simulink subsystem "window_control"  (R2021b)
settings: Solver=VariableStepAuto  StartTime=0.0  StopTime=10.0  RelTol=1e-3
values from neighbouring files (symbols this model uses):
  armature_position = Simulink.Parameter    [Parameters.m]
  energy_save_speed = Simulink.Parameter    [Parameters.m]
  window_speed = Simulink.Parameter    [Parameters.m]
libraries: simulink x1
settings Model: Creator=Mindmotiv  LastModifiedBy=wiechowski
settings SolverCC: AlgebraicLoopSolver=TrustRegion
settings DebuggingCC: SFMachineParentedDataDiag=warning

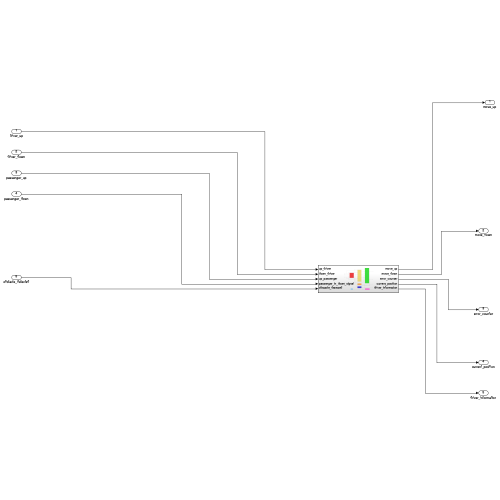
[thumbnail: Simulink's stored preview of the top-level diagram]
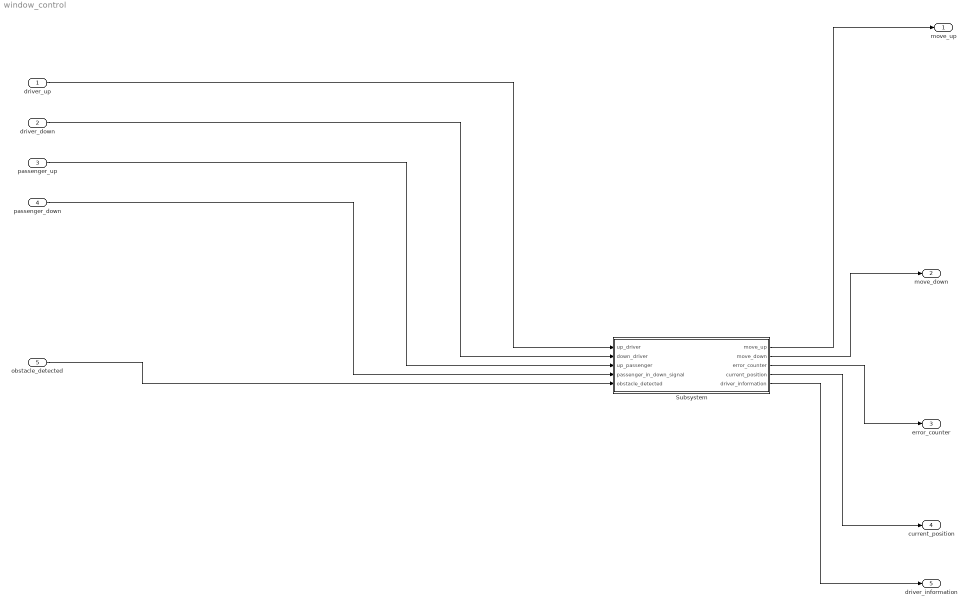
== system window_control ==
  driver_up : Inport
  driver_down : Inport  Port=2
  passenger_up : Inport  Port=3
  passenger_down : Inport  Port=4
  obstacle_detected : Inport  Port=5
  Subsystem : Subsystem
  move_up : Outport
  move_down : Outport  Port=2
  error_counter : Outport  Port=3
  current_position : Outport  Port=4
  driver_information : Outport  Port=5
  wires:
  driver_up/1 -> Subsystem/1(up_driver)
  driver_down/1 -> Subsystem/2(down_driver)
  passenger_up/1 -> Subsystem/3(up_passenger)
  passenger_down/1 -> Subsystem/4(passenger_in_down_signal)
  obstacle_detected/1 -> Subsystem/5(obstacle_detected)
  Subsystem/1(move_up) -> move_up/1
  Subsystem/2(move_down) -> move_down/1
  Subsystem/3(error_counter) -> error_counter/1
  Subsystem/4(current_position) -> current_position/1
  Subsystem/5(driver_information) -> driver_information/1

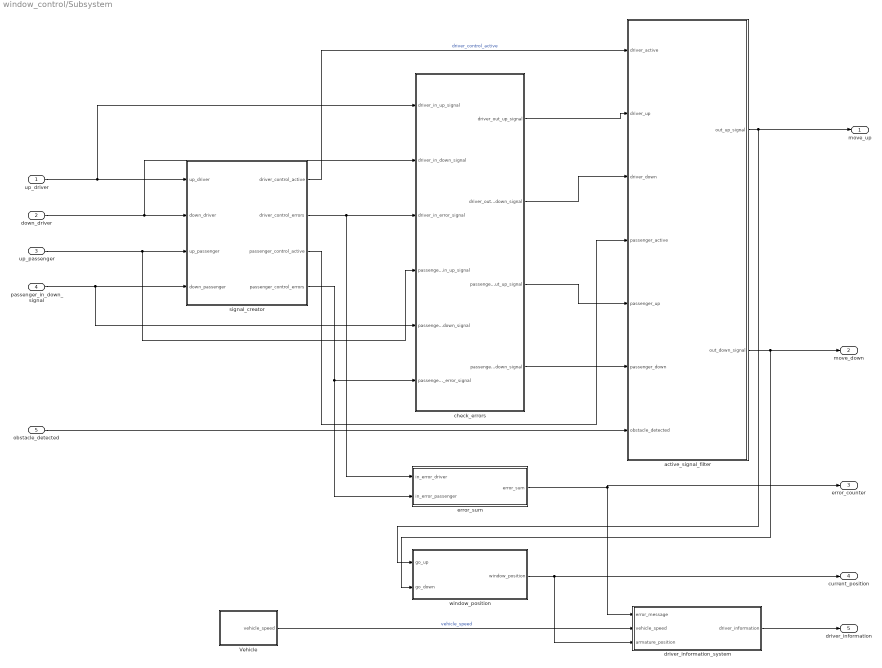
== system window_control/Subsystem ==
  up_driver : Inport
  down_driver : Inport  Port=2
  up_passenger : Inport  Port=3
  passenger_in_down_signal : Inport  Port=4
  obstacle_detected : Inport  Port=5
  Vehicle : Subsystem
  active_signal_filter : Subsystem
  check_errors : Subsystem
  driver_information_system : Subsystem
  error_sum : Subsystem
  signal_creator : Subsystem
  window_position : Subsystem
  move_up : Outport
  move_down : Outport  Port=2
  error_counter : Outport  Port=3
  current_position : Outport  Port=4
  driver_information : Outport  Port=5
  wires:
  obstacle_detected/1 -> active_signal_filter/7(obstacle_detected)
  check_errors/2(driver_out_down_signal) -> active_signal_filter/3(driver_down)
  driver_information_system/1(driver_information) -> driver_information/1
  Vehicle/1(vehicle_speed) -> driver_information_system/2(vehicle_speed)  "vehicle_speed"
  signal_creator/3(passenger_control_active) -> active_signal_filter/4(passenger_active)
  signal_creator/1(driver_control_active) -> active_signal_filter/1(driver_active)  "driver_control_active"
  check_errors/3(passenger_out_up_signal) -> active_signal_filter/5(passenger_up)
  check_errors/4(passenger_out_down_signal) -> active_signal_filter/6(passenger_down)
  up_passenger/1 -> signal_creator/3(up_passenger), check_errors/4(passenger_in_up_signal)
  window_position/1(window_position) -> current_position/1, driver_information_system/3(armature_position)
  up_driver/1 -> signal_creator/1(up_driver), check_errors/1(driver_in_up_signal)
  down_driver/1 -> signal_creator/2(down_driver), check_errors/2(driver_in_down_signal)
  signal_creator/4(passenger_control_errors) -> check_errors/6(passenger_in_error_signal), error_sum/2(in_error_passenger)
  passenger_in_down_signal/1 -> check_errors/5(passenger_in_down_signal), signal_creator/4(down_passenger)
  signal_creator/2(driver_control_errors) -> check_errors/3(driver_in_error_signal), error_sum/1(in_error_driver)
  active_signal_filter/1(out_up_signal) -> move_up/1, window_position/1(go_up)
  check_errors/1(driver_out_up_signal) -> active_signal_filter/2(driver_up)
  active_signal_filter/2(out_down_signal) -> move_down/1, window_position/2(go_down)
  error_sum/1(error_sum) -> error_counter/1, driver_information_system/1(error_message)

== system window_control/Subsystem/Vehicle ==
  Constant : Constant  Value=0
  vehicle_speed : Outport
  wires:
  Constant/1 -> vehicle_speed/1

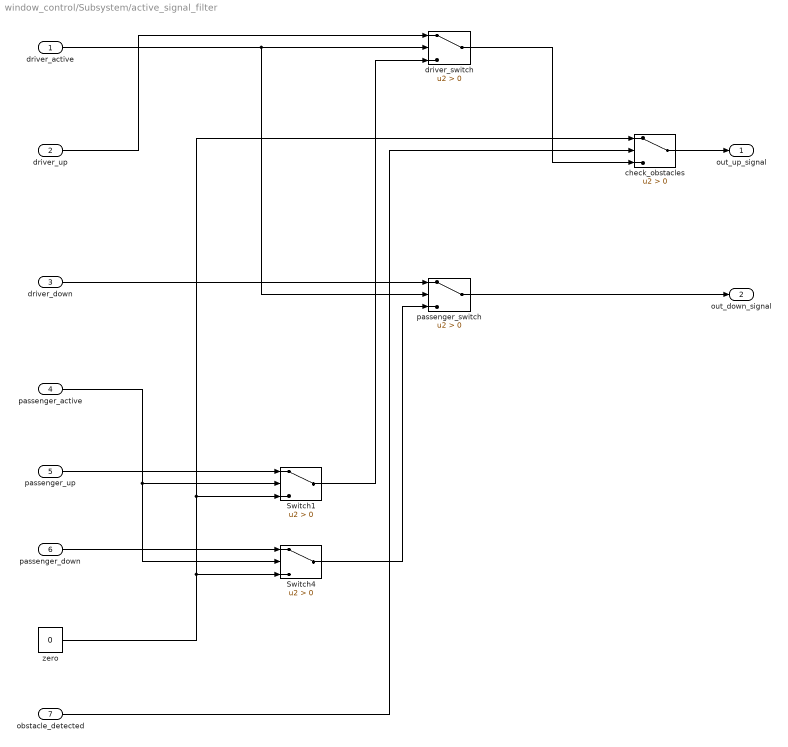
== system window_control/Subsystem/active_signal_filter ==
  driver_active : Inport
  driver_up : Inport  Port=2
  driver_down : Inport  Port=3
  passenger_active : Inport  Port=4
  passenger_up : Inport  Port=5
  passenger_down : Inport  Port=6
  obstacle_detected : Inport  Port=7
  Switch1 : Switch  Criteria=u2 > Threshold
  Switch4 : Switch  Criteria=u2 > Threshold
  check_obstacles : Switch  Criteria=u2 > Threshold
  driver_switch : Switch  Criteria=u2 > Threshold
  passenger_switch : Switch  Criteria=u2 > Threshold
  zero : Constant  Value=0
  out_up_signal : Outport
  out_down_signal : Outport  Port=2
  wires:
  check_obstacles/1 -> out_up_signal/1
  driver_switch/1 -> check_obstacles/3
  obstacle_detected/1 -> check_obstacles/2
  passenger_switch/1 -> out_down_signal/1
  Switch4/1 -> passenger_switch/3
  passenger_down/1 -> Switch4/1
  driver_down/1 -> passenger_switch/1
  passenger_up/1 -> Switch1/1
  Switch1/1 -> driver_switch/3
  passenger_active/1 -> Switch1/2, Switch4/2
  driver_up/1 -> driver_switch/1
  zero/1 -> Switch1/3, check_obstacles/1, Switch4/3
  driver_active/1 -> driver_switch/2, passenger_switch/2

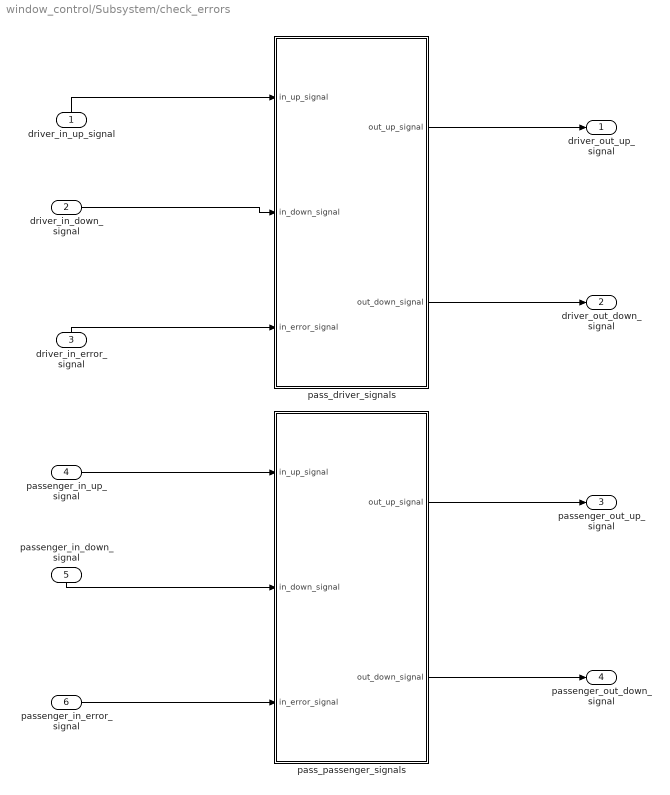
== system window_control/Subsystem/check_errors ==
  driver_in_up_signal : Inport
  driver_in_down_signal : Inport  Port=2
  driver_in_error_signal : Inport  Port=3
  passenger_in_up_signal : Inport  Port=4
  passenger_in_down_signal : Inport  Port=5
  passenger_in_error_signal : Inport  Port=6
  pass_driver_signals : Subsystem
  pass_passenger_signals : Subsystem
  driver_out_up_signal : Outport
  driver_out_down_signal : Outport  Port=2
  passenger_out_up_signal : Outport  Port=3
  passenger_out_down_signal : Outport  Port=4
  wires:
  driver_in_error_signal/1 -> pass_driver_signals/3(in_error_signal)
  pass_driver_signals/2(out_down_signal) -> driver_out_down_signal/1
  pass_driver_signals/1(out_up_signal) -> driver_out_up_signal/1
  passenger_in_error_signal/1 -> pass_passenger_signals/3(in_error_signal)
  passenger_in_down_signal/1 -> pass_passenger_signals/2(in_down_signal)
  driver_in_down_signal/1 -> pass_driver_signals/2(in_down_signal)
  passenger_in_up_signal/1 -> pass_passenger_signals/1(in_up_signal)
  pass_passenger_signals/1(out_up_signal) -> passenger_out_up_signal/1
  driver_in_up_signal/1 -> pass_driver_signals/1(in_up_signal)
  pass_passenger_signals/2(out_down_signal) -> passenger_out_down_signal/1

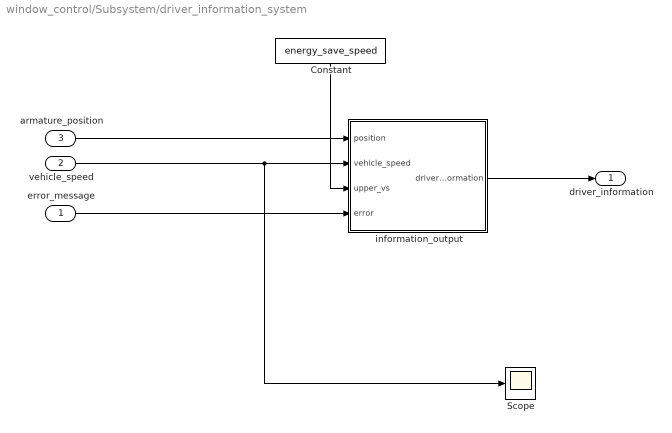
== system window_control/Subsystem/driver_information_system ==
  error_message : Inport
  vehicle_speed : Inport  Port=2
  armature_position : Inport  Port=3
  Constant : Constant  Value=energy_save_speed
  Scope : Scope
  information_output : MATLAB Function  TreatAsAtomicUnit=on
  driver_information : Outport
  wires:
  armature_position/1 -> information_output/1(position)
  information_output/1(driver_information) -> driver_information/1
  vehicle_speed/1 -> information_output/2(vehicle_speed), Scope/1
  error_message/1 -> information_output/4(error)
  Constant/1 -> information_output/3(upper_vs)

== system window_control/Subsystem/error_sum ==
  in_error_driver : Inport
  in_error_passenger : Inport  Port=2
  Add : Sum
  error_sum : Outport
  wires:
  in_error_driver/1 -> Add/1
  in_error_passenger/1 -> Add/2
  Add/1 -> error_sum/1

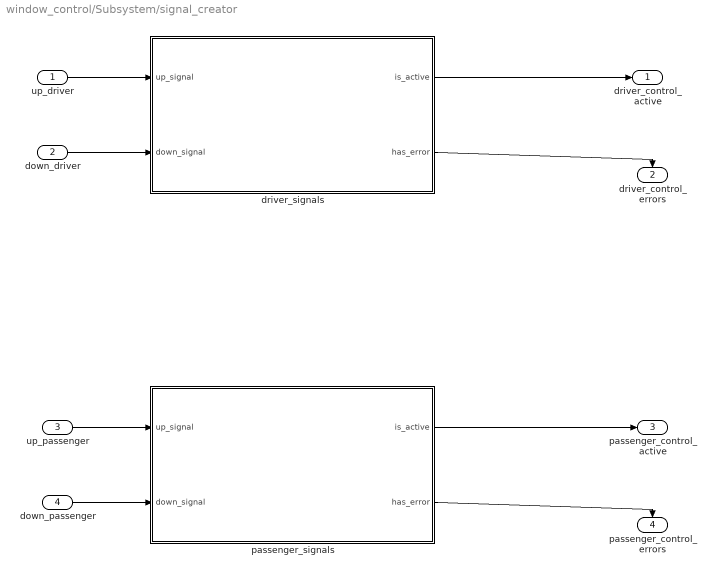
== system window_control/Subsystem/signal_creator ==
  up_driver : Inport
  down_driver : Inport  Port=2
  up_passenger : Inport  Port=3
  down_passenger : Inport  Port=4
  driver_signals : Subsystem
  passenger_signals : Subsystem
  driver_control_active : Outport
  driver_control_errors : Outport  Port=2
  passenger_control_active : Outport  Port=3
  passenger_control_errors : Outport  Port=4
  wires:
  up_passenger/1 -> passenger_signals/1(up_signal)
  up_driver/1 -> driver_signals/1(up_signal)
  down_passenger/1 -> passenger_signals/2(down_signal)
  passenger_signals/2(has_error) -> passenger_control_errors/1
  down_driver/1 -> driver_signals/2(down_signal)
  passenger_signals/1(is_active) -> passenger_control_active/1
  driver_signals/2(has_error) -> driver_control_errors/1
  driver_signals/1(is_active) -> driver_control_active/1

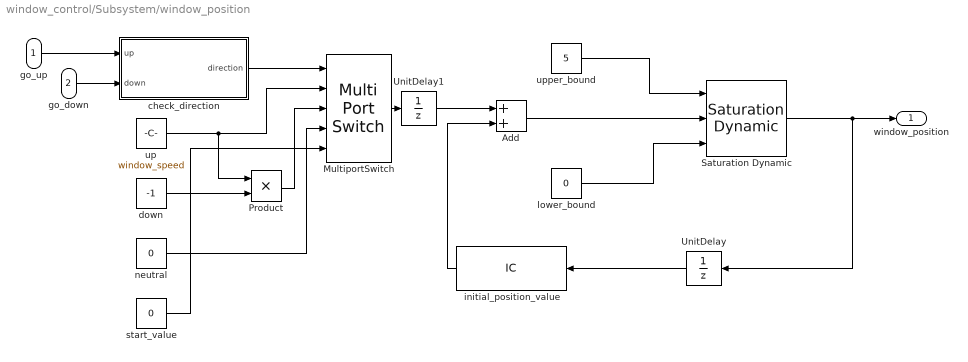
== system window_control/Subsystem/window_position ==
  go_up : Inport
  go_down : Inport  Port=2
  Add : Sum
  MultiportSwitch : MultiPortSwitch  DataPortOrder=Zero-based contiguous  Inputs=4  zeroidx=on
  Product : Product  RndMeth=Zero
  Saturation Dynamic : simulink/Discontinuities/Saturation Dynamic  OutMin=0  OutMax=100  OutDataTypeStr=Inherit: Same as second input  OutDataType=fixdt(1, 16)  OutScaling=2^-10  DoSatur=off
  UnitDelay : UnitDelay  SampleTime=-1  HasFrameUpgradeWarning=on
  UnitDelay1 : UnitDelay  SampleTime=-1  HasFrameUpgradeWarning=on
  check_direction : MATLAB Function  TreatAsAtomicUnit=on
  down : Constant  Value=-1
  initial_position_value : InitialCondition  Value=armature_position
  lower_bound : Constant  Value=0
  neutral : Constant  Value=0
  start_value : Constant  Value=0
  up : Constant  Value=window_speed
  upper_bound : Constant  Value=5
  window_position : Outport
  wires:
  UnitDelay1/1 -> Add/1
  Product/1 -> MultiportSwitch/3
  Add/1 -> Saturation Dynamic/2
  up/1 -> MultiportSwitch/2, Product/1
  start_value/1 -> MultiportSwitch/5
  Saturation Dynamic/1 -> window_position/1, UnitDelay/1
  check_direction/1(direction) -> MultiportSwitch/1
  down/1 -> Product/2
  neutral/1 -> MultiportSwitch/4
  MultiportSwitch/1 -> UnitDelay1/1
  go_up/1 -> check_direction/1(up)
  UnitDelay/1 -> initial_position_value/1
  lower_bound/1 -> Saturation Dynamic/3
  go_down/1 -> check_direction/2(down)
  initial_position_value/1 -> Add/2
  upper_bound/1 -> Saturation Dynamic/1

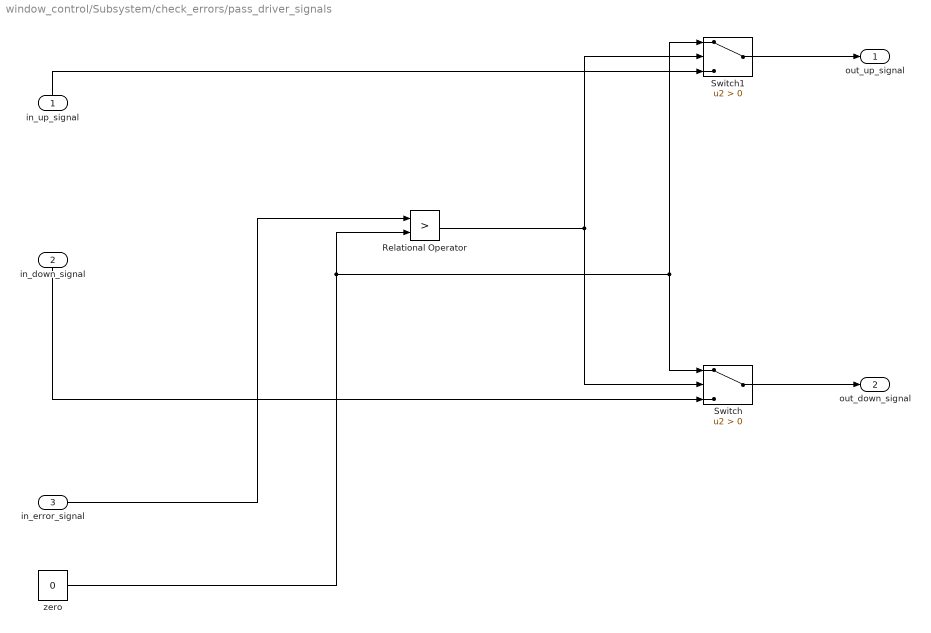
== system window_control/Subsystem/check_errors/pass_driver_signals ==
  in_up_signal : Inport
  in_down_signal : Inport  Port=2
  in_error_signal : Inport  Port=3
  Relational Operator : RelationalOperator  Operator=>  OutDataTypeStr=boolean  RndMeth=Nearest
  Switch : Switch  Criteria=u2 > Threshold
  Switch1 : Switch  Criteria=u2 > Threshold
  zero : Constant  Value=0
  out_up_signal : Outport
  out_down_signal : Outport  Port=2
  wires:
  Relational Operator/1 -> Switch/2, Switch1/2
  Switch/1 -> out_down_signal/1
  zero/1 -> Relational Operator/2, Switch/1, Switch1/1
  in_error_signal/1 -> Relational Operator/1
  in_down_signal/1 -> Switch/3
  in_up_signal/1 -> Switch1/3
  Switch1/1 -> out_up_signal/1

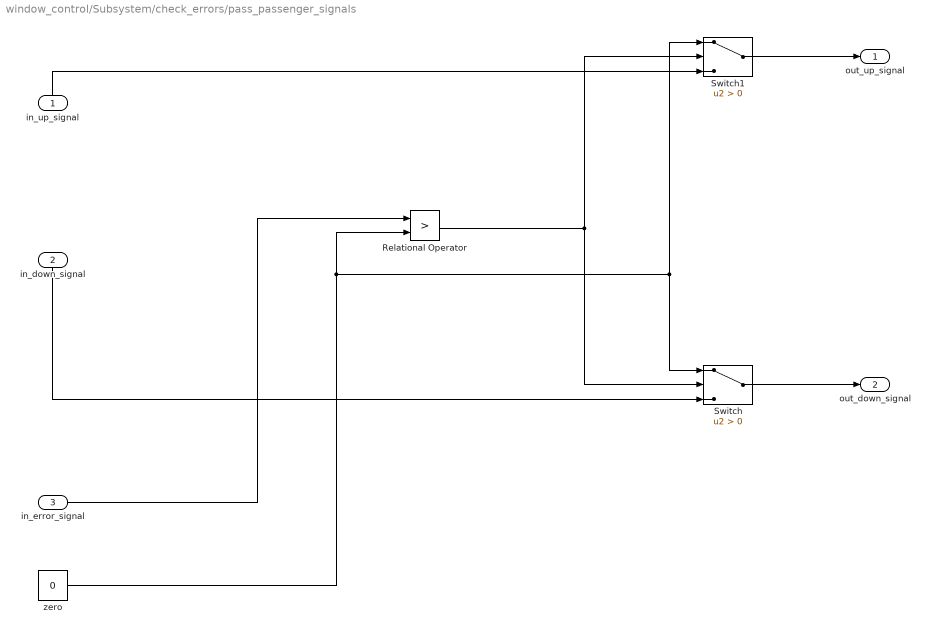
== system window_control/Subsystem/check_errors/pass_passenger_signals ==
  in_up_signal : Inport
  in_down_signal : Inport  Port=2
  in_error_signal : Inport  Port=3
  Relational Operator : RelationalOperator  Operator=>  OutDataTypeStr=boolean  RndMeth=Nearest
  Switch : Switch  Criteria=u2 > Threshold
  Switch1 : Switch  Criteria=u2 > Threshold
  zero : Constant  Value=0
  out_up_signal : Outport
  out_down_signal : Outport  Port=2
  wires:
  Relational Operator/1 -> Switch/2, Switch1/2
  Switch/1 -> out_down_signal/1
  zero/1 -> Relational Operator/2, Switch/1, Switch1/1
  in_error_signal/1 -> Relational Operator/1
  in_down_signal/1 -> Switch/3
  in_up_signal/1 -> Switch1/3
  Switch1/1 -> out_up_signal/1

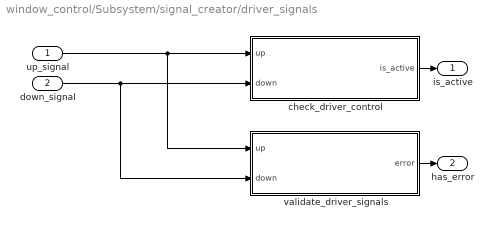
== system window_control/Subsystem/signal_creator/driver_signals ==
  up_signal : Inport
  down_signal : Inport  Port=2
  check_driver_control : Subsystem
  validate_driver_signals : Subsystem
  is_active : Outport
  has_error : Outport  Port=2
  wires:
  down_signal/1 -> check_driver_control/2(down), validate_driver_signals/2(down)
  up_signal/1 -> check_driver_control/1(up), validate_driver_signals/1(up)
  validate_driver_signals/1(error) -> has_error/1
  check_driver_control/1(is_active) -> is_active/1

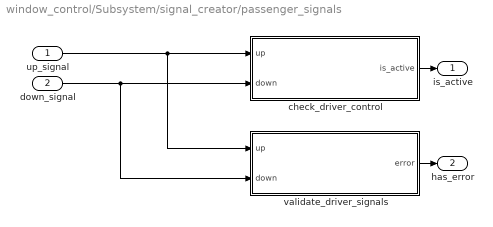
== system window_control/Subsystem/signal_creator/passenger_signals ==
  up_signal : Inport
  down_signal : Inport  Port=2
  check_driver_control : Subsystem
  validate_driver_signals : Subsystem
  is_active : Outport
  has_error : Outport  Port=2
  wires:
  down_signal/1 -> check_driver_control/2(down), validate_driver_signals/2(down)
  up_signal/1 -> check_driver_control/1(up), validate_driver_signals/1(up)
  validate_driver_signals/1(error) -> has_error/1
  check_driver_control/1(is_active) -> is_active/1

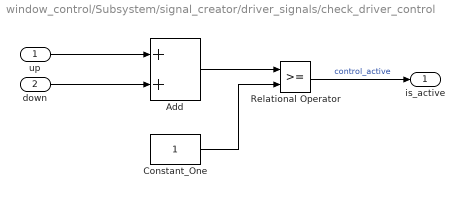
== system window_control/Subsystem/signal_creator/driver_signals/check_driver_control ==
  up : Inport
  down : Inport  Port=2
  Add : Sum
  Constant_One : Constant
  Relational Operator : RelationalOperator  OutDataTypeStr=boolean  RndMeth=Nearest
  is_active : Outport
  wires:
  up/1 -> Add/1
  down/1 -> Add/2
  Add/1 -> Relational Operator/1
  Relational Operator/1 -> is_active/1  "control_active"
  Constant_One/1 -> Relational Operator/2

== system window_control/Subsystem/signal_creator/driver_signals/validate_driver_signals ==
  up : Inport
  down : Inport  Port=2
  Add : Sum
  Relational Operator : RelationalOperator  OutDataTypeStr=boolean  RndMeth=Nearest
  two : Constant  Value=2
  error : Outport
  wires:
  up/1 -> Add/1
  down/1 -> Add/2
  Add/1 -> Relational Operator/1
  Relational Operator/1 -> error/1  "error_signal"
  two/1 -> Relational Operator/2

== system window_control/Subsystem/signal_creator/passenger_signals/check_driver_control ==
  up : Inport
  down : Inport  Port=2
  Add : Sum
  Constant_One : Constant
  Relational Operator : RelationalOperator  OutDataTypeStr=boolean  RndMeth=Nearest
  is_active : Outport
  wires:
  up/1 -> Add/1
  down/1 -> Add/2
  Add/1 -> Relational Operator/1
  Relational Operator/1 -> is_active/1  "control_active"
  Constant_One/1 -> Relational Operator/2

== system window_control/Subsystem/signal_creator/passenger_signals/validate_driver_signals ==
  up : Inport
  down : Inport  Port=2
  Add : Sum
  Relational Operator : RelationalOperator  OutDataTypeStr=boolean  RndMeth=Nearest
  two : Constant  Value=2
  error : Outport
  wires:
  up/1 -> Add/1
  down/1 -> Add/2
  Add/1 -> Relational Operator/1
  Relational Operator/1 -> error/1  "error_signal"
  two/1 -> Relational Operator/2

== matlab function window_control/Subsystem/driver_information_system/information_output ==
  data: position input; vehicle_speed input; driver_information output; upper_vs input; error input
function driver_information = fcn(position, vehicle_speed, upper_vs, error)
%#codegen

%everything is ok
driver_information = 0;
if error>0
    %at least one error occured
    driver_information = 2;
elseif vehicle_speed >= upper_vs
    %window should close to save energy if it is open and the speed is high
    if position < 100
        driver_information = 1;
    end   
end

== matlab function window_control/Subsystem/window_position/check_direction ==
  data: up input; direction output; down input
function direction = fcn(up,down)
%#codegen

if up == 1
    direction = 0;
elseif down == 1
        direction = 1;
else
    direction = 2;
end
